simulink model "CC_CV"  (R2019a)
settings: Solver=ode23s  StartTime=0.0  StopTime=99  FixedStep=50e-6  RelTol=1e-8
libraries: powerlib x10, simulink x8
settings Model: Creator=Soto Porras  LastModifiedBy=juanj
settings DataIOCC: ReturnWorkspaceOutputs=off
settings DebuggingCC: ArithmeticOperatorsInVariantConditions=warning

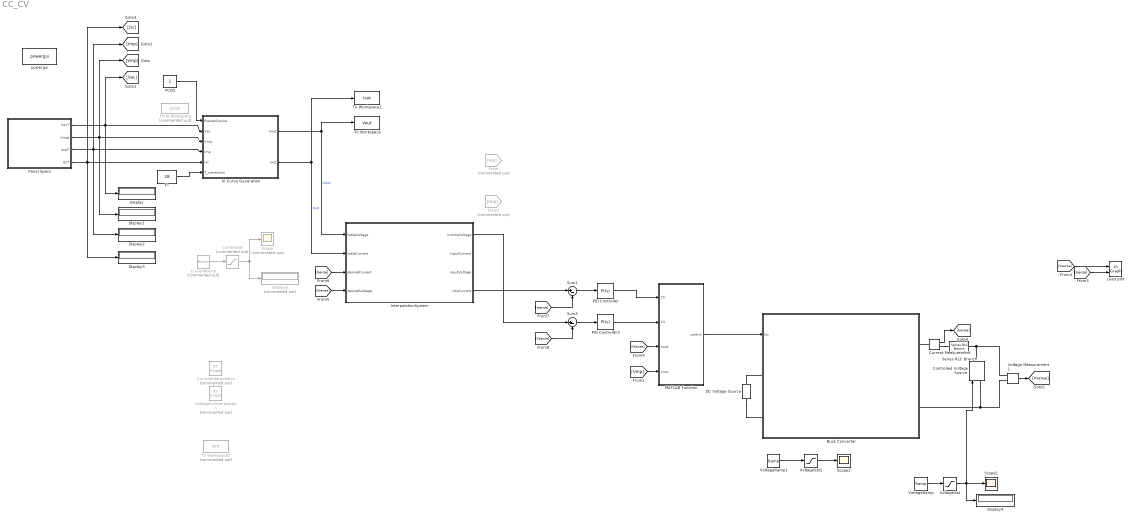
== system CC_CV ==
  Buck Converter : Subsystem
  Controlled Voltage Source : powerlib/Electrical Sources/Controlled Voltage Source  Initialize=off  Source_Type=DC  Amplitude=0  Phase=0  Frequency=0  Measurements=None
      settings: SourceProductName=Simscape Electrical
  Current Measurement : powerlib/Measurements/Current Measurement  PhasorSimulation=off  OutputType=Complex  PSBequivalent=0
      settings: SourceProductName=Simscape Electrical
  CurrentInterpolation : simulink/Sinks/XY Graph  Commented=on  xmin=0  xmax=6  ymin=0  ymax=2  st=-1
  CurrentRamp : simulink/Sources/Ramp  Commented=on  slope=0.015603  start=0  InitialOutput=0
  CurrentSat : Saturate  Commented=on  UpperLimit=1.5603  LowerLimit=0
  DC Voltage Source : powerlib/Electrical Sources/DC Voltage Source  Amplitude=15  Measurements=None
      settings: SourceProductName=Simscape Electrical
  Display{,1..4} (5 alike) : Display
  Display5 : Display  Commented=on
  From : From  Commented=on  GotoTag=Voc
  From Workspace : FromWorkspace  Commented=on  VariableName=pcos  SampleTime=0
  From2 : From  Commented=on  GotoTag=Imp
  IV Curve Generation : Subsystem  mask(Panel I-V Curve Calculation){ValueVocComp=0.0062, ValueVmpComp=0.0067}
      mask prompts: ValueVocComp "Voc Temperature Correction (V)"; ValueVmpComp "Vmp Temperature Correction (V)"
      mask help:
      | This module calculates the panel IV curve using the next panel parameters:
      | 1. Voc
      | 2. Vmp
      | 3. Imp
      | 4. Isc
      |
      | It applies:
      | 1. Correction to current parameters (Isc and Imp) using a pseudo cosine that varies depending on the angle of the perpendicular CubeSat face and the sun's incident radiation.
      | 2. Correction to voltage parameters (Voc and Vmp) using the panel datasheet voltage losses, given in V by the user.
      mask TypeOptions ValueVocComp: Voc_comp/Value
      mask TypeOptions ValueVmpComp: Vmp_comp/Value
      mask Display: image('IV_curve.png');
  InterpolationSystem : Subsystem
  Load plot : simulink/Sinks/XY Graph  xmin=0  xmax=6  ymin=0  ymax=2  st=-1
  MATLAB Function : MATLAB Function  TreatAsAtomicUnit=on
  PCOS : Constant
  PID Controller : simulink/Continuous/PID Controller  Controller=PI  Form=Parallel  TimeDomain=Continuous-time  SampleTime=0.00005  IntegratorMethod=Trapezoidal  FilterMethod=Forward Euler  ControllerParametersSource=internal  P=20  I=0.5  D=0  UseFilter=on  N=100  TunerSelectOption=Frequency Response Based  InitialConditionSource=internal  InitialConditionForIntegrator=0  InitialConditionForFilter=0  DifferentiatorICPrevScaledInput=0  ExternalReset=none  TrackingMode=off  Kt=1  LimitOutput=off  UpperSaturationLimit=inf  LowerSaturationLimit=-inf  LinearizeAsGain=on  AntiWindupMode=none  Kb=1  POutMin=[]  POutMax=[]  IOutMin=[]  IOutMax=[]  DOutMin=[]  DOutMax=[]  NOutMin=[]  NOutMax=[]  SumOutMin=[]  SumOutMax=[]  SaturationOutMin=[]  SaturationOutMax=[]  PParamMin=[]  PParamMax=[]  IParamMin=[]  IParamMax=[]  DParamMin=[]  DParamMax=[]  NParamMin=[]  NParamMax=[]  KbParamMin=[]  KbParamMax=[]  KtParamMin=[]  KtParamMax=[]  KbOutMin=[]  KbOutMax=[]  KtOutMin=[]  KtOutMax=[]  IntegratorOutMin=[]  IntegratorOutMax=[]  FilterOutMin=[]  FilterOutMax=[]  SumI1OutMin=[]  SumI1OutMax=[]  SumI2OutMin=[]  SumI2OutMax=[]  SumI3OutMin=[]  SumI3OutMax=[]  SumI4OutMin=[]  SumI4OutMax=[]  SumDOutMin=[]  SumDOutMax=[]  DifferentiatorOutMin=[]  DifferentiatorOutMax=[]  FilterDiffOutCoefMin=[]  FilterDiffOutCoefMax=[]  ReciprocalOutMin=[]  ReciprocalOutMax=[]  SumDenOutMin=[]  SumDenOutMax=[]  SumNumOutMin=[]  SumNumOutMax=[]  DivideOutMin=[]  DivideOutMax=[]  IntegratorContinuousStateAttributes=''  IntegratorStateMustResolveToSignalObject=off  IntegratorRTWStateStorageClass=Auto  FilterContinuousStateAttributes=''  FilterStateMustResolveToSignalObject=off  FilterRTWStateStorageClass=Auto  ParallelPVariant=InternalParameters  IdealPVariant=Disabled  IVariant=InternalParameters  DVariant=Disabled  IntegratorVariant=Continuous  SatVariant=Disabled  AWVariant=Passthrough  PCopyVariant=Disabled  TRVariant=Disabled  FdbkBlocksVariant=Forward  IdealPFdbkVariant=Disabled  SatFdbkVariant=Disabled  DerivativeFilterVariant=Disabled  NVariant=Disabled  NCopyVariant=Disabled_SignalSpec  FilterICVariant=Disabled  IntegratorICVariant=InternalICs  ExternalResetVariant=Disabled  TRSumVariant=Passthrough  SumFdbkVariant=Disabled  SumVariant=Sum_PI
  PID Controller2 : simulink/Continuous/PID Controller  Controller=PI  Form=Parallel  TimeDomain=Continuous-time  SampleTime=0.00005  IntegratorMethod=Trapezoidal  FilterMethod=Forward Euler  ControllerParametersSource=internal  P=20  I=0.01  D=0  UseFilter=on  N=100  TunerSelectOption=Frequency Response Based  InitialConditionSource=internal  InitialConditionForIntegrator=0  InitialConditionForFilter=0  DifferentiatorICPrevScaledInput=0  ExternalReset=none  TrackingMode=off  Kt=1  LimitOutput=off  UpperSaturationLimit=inf  LowerSaturationLimit=-inf  LinearizeAsGain=on  AntiWindupMode=none  Kb=1  POutMin=[]  POutMax=[]  IOutMin=[]  IOutMax=[]  DOutMin=[]  DOutMax=[]  NOutMin=[]  NOutMax=[]  SumOutMin=[]  SumOutMax=[]  SaturationOutMin=[]  SaturationOutMax=[]  PParamMin=[]  PParamMax=[]  IParamMin=[]  IParamMax=[]  DParamMin=[]  DParamMax=[]  NParamMin=[]  NParamMax=[]  KbParamMin=[]  KbParamMax=[]  KtParamMin=[]  KtParamMax=[]  KbOutMin=[]  KbOutMax=[]  KtOutMin=[]  KtOutMax=[]  IntegratorOutMin=[]  IntegratorOutMax=[]  FilterOutMin=[]  FilterOutMax=[]  SumI1OutMin=[]  SumI1OutMax=[]  SumI2OutMin=[]  SumI2OutMax=[]  SumI3OutMin=[]  SumI3OutMax=[]  SumI4OutMin=[]  SumI4OutMax=[]  SumDOutMin=[]  SumDOutMax=[]  DifferentiatorOutMin=[]  DifferentiatorOutMax=[]  FilterDiffOutCoefMin=[]  FilterDiffOutCoefMax=[]  ReciprocalOutMin=[]  ReciprocalOutMax=[]  SumDenOutMin=[]  SumDenOutMax=[]  SumNumOutMin=[]  SumNumOutMax=[]  DivideOutMin=[]  DivideOutMax=[]  IntegratorContinuousStateAttributes=''  IntegratorStateMustResolveToSignalObject=off  IntegratorRTWStateStorageClass=Auto  FilterContinuousStateAttributes=''  FilterStateMustResolveToSignalObject=off  FilterRTWStateStorageClass=Auto  ParallelPVariant=InternalParameters  IdealPVariant=Disabled  IVariant=InternalParameters  DVariant=Disabled  IntegratorVariant=Continuous  SatVariant=Disabled  AWVariant=Passthrough  PCopyVariant=Disabled  TRVariant=Disabled  FdbkBlocksVariant=Forward  IdealPFdbkVariant=Disabled  SatFdbkVariant=Disabled  DerivativeFilterVariant=Disabled  NVariant=Disabled  NCopyVariant=Disabled_SignalSpec  FilterICVariant=Disabled  IntegratorICVariant=InternalICs  ExternalResetVariant=Disabled  TRSumVariant=Passthrough  SumFdbkVariant=Disabled  SumVariant=Sum_PI
  Panel Specs : Subsystem  mask(Solar Panel Specifications){Voc=2.690, Vmp=2.409, Imp=0.5029, Isc=0.5196, SerialGain=2, ParallelGain=3}
      mask prompts: SerialGain "Serial"; ParallelGain "Parallel"
      mask help: Inputs solar panel electrical specifications, temperature and array distribution.
      mask TypeOptions Voc: Voc/Value
      mask TypeOptions Vmp: Vmp/Value
      mask TypeOptions Imp: Imp/Value
      mask TypeOptions Isc: Isc/Value
      mask TypeOptions SerialGain: Gain/Gain | Gain1/Gain
      mask TypeOptions ParallelGain: Gain2/Gain | Gain3/Gain
      mask DialogControl Container3 Prompt: Panel Array
      mask Display: image('solar_panel.png');
  Scope : Scope  Commented=on
  Scope1 : Scope
  Scope2 : Scope
  Series RLC Branch : powerlib/Elements/Series RLC Branch  LConnTagsString=__new0  RConnTagsString=__new0  BranchType=R  Resistance=1e-5  Inductance=1e-3  SetiL0=off  InitialCurrent=0  Capacitance=1e-6  Setx0=off  InitialVoltage=0  Measurements=None
      settings: SourceProductName=Simscape Electrical
  Sum1 : Sum  Inputs=|+-
  Sum3 : Sum  Inputs=|+-
  To Workspace : ToWorkspace  VariableName=Vout  SaveFormat=Structure With Time  SampleTime=-1
  To Workspace1 : ToWorkspace  VariableName=Iout  SaveFormat=Structure With Time  SampleTime=-1
  To Workspace2 : ToWorkspace  Commented=on  VariableName=Vint  SaveFormat=Structure With Time  SampleTime=-1
  T° : Constant  Value=28
  Voltage Measurement1 : powerlib/Measurements/Voltage Measurement  PhasorSimulation=off  OutputType=Complex  PSBequivalent=0
      settings: SourceProductName=Simscape Electrical
  VoltageInvInterpolation : simulink/Sinks/XY Graph  Commented=on  xmin=0  xmax=6  ymin=0  ymax=2  st=-1
  VoltageRamp : simulink/Sources/Ramp  slope=0.0538  start=0  InitialOutput=0
  VoltageRamp1 : simulink/Sources/Ramp  slope=0.0538  start=0  InitialOutput=0
  VoltageSat : Saturate  UpperLimit=5.37  LowerLimit=0.1
  VoltageSat1 : Saturate  UpperLimit=5.38  LowerLimit=0.1
  powergui : powerlib/powergui  Priority=1  SimulationMode=Continuous  SampleTime=50e-6  frequency=60  Iterations=50  frequencyindice=0  Pbase=100e6  ErrMax=1e-4  UnitsV=kV  UnitsW=MW  buscounter=0  FunctionMessages=off  echomessages=off  EnableUseOfTLC=off  CurrentSourceSwitches=off  DisableSnubberDevices=off  DisableRonSwitches=off  DisableVfSwitches=off  DisplayEquations=off  AutomaticDiscreteSolvers=off  SolverType=Tustin/Backward Euler (TBE)  Interpol=off  ExternalGateDelay=off  methode=off  Ts=100  x0status=blocks  SPID=on  SwTol=0  HookPort=off  NonlinearTolerance=0  nMaxIteration=15  ContinueOnMaxIteration=off  RestoreLinks=warning  ResistiveCurrentMeasurement=off  Frange=[0:2:500]  Ylog=off  Xlog=on  ShowGrid=off  save=off  variable=ZData  structure=0  ZoomFFT=off  StartTime=0.0  cycles=1  DisplayStyle=1  fundamental=60  FreqAxis=off  MaxFrequency=1000  frequencyindicesteady=1  RmsSteady=1  display=off
      settings: SourceProductName=Simscape Electrical
  wires:
  Panel Specs/1(VocT) -> [Voc], Display/1, IV Curve Generation/2(Voc)
  Panel Specs/2(Vmpt) -> [Vmp], Display1/1, IV Curve Generation/3(Vmp)
  Panel Specs/3(ImpT) -> [Imp], Display2/1, IV Curve Generation/4(Imp)
  Panel Specs/4(IscT) -> [Isc], Display3/1, IV Curve Generation/5(Isc)
  CurrentRamp/1 -> CurrentSat/1
  IV Curve Generation/1(Vout) -> InterpolationSystem/1(tableVoltage), To Workspace/1  "Vout"
  IV Curve Generation/2(Iout) -> To Workspace1/1, InterpolationSystem/2(tableCurrent)  "Iout"
  CurrentSat/1 -> Display5/1, Scope/1
  T°/1 -> IV Curve Generation/6(T_correction)
  Sum1/1 -> PID Controller/1
  VoltageRamp/1 -> VoltageSat/1
  VoltageSat/1 -> Controlled Voltage Source/1, Scope1/1, Display4/1
  Voltage Measurement1/1 -> [Vsense]
  Current Measurement/1 -> [Isense]
  VoltageRamp1/1 -> VoltageSat1/1
  VoltageSat1/1 -> Scope2/1
  InterpolationSystem/4(intpCurrent) -> Sum1/1
  PID Controller/1 -> MATLAB Function/1(CC)
  MATLAB Function/1(control) -> Buck Converter/1(Dc)
  PID Controller2/1 -> MATLAB Function/2(CV)
  Sum3/1 -> PID Controller2/1
  InterpolationSystem/1(invIntpVoltage) -> Sum3/1
  [Isense] -> Load plot/2
  [Vsense] -> Load plot/1
  [Vsense] -> InterpolationSystem/4(desiredVotlage)
  [Isense] -> InterpolationSystem/3(desiredCurrent)
  [Isense] -> Sum1/2
  [Vsense] -> Sum3/2
  [Vsense] -> MATLAB Function/3(Vout)
  [Vmp] -> MATLAB Function/4(Vmp)
  PCOS/1 -> IV Curve Generation/1(PseudoCosine)
  connections:
  DC Voltage Source/RConn1 -- Buck Converter/LConn1
  DC Voltage Source/LConn1 -- Buck Converter/LConn2
  Voltage Measurement1/LConn2 -- Controlled Voltage Source/LConn1 -- Buck Converter/RConn2
  Series RLC Branch/LConn1 -- Voltage Measurement1/LConn1 -- Controlled Voltage Source/RConn1
  Current Measurement/LConn1 -- Buck Converter/RConn1
  Current Measurement/RConn1 -- Series RLC Branch/RConn1

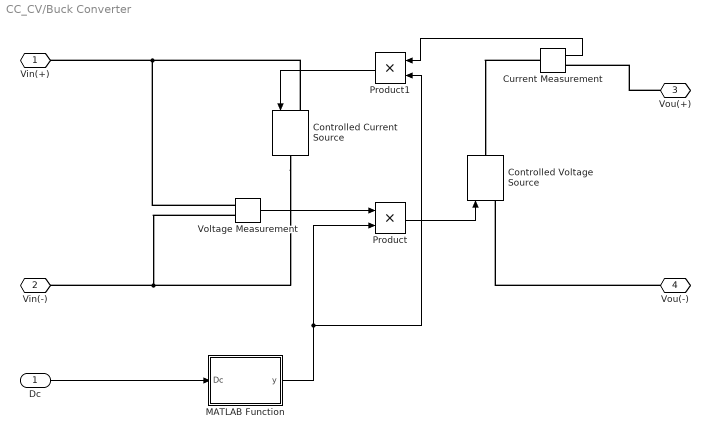
== system CC_CV/Buck Converter ==
  Dc : Inport
  Controlled Current Source : powerlib/Electrical Sources/Controlled Current Source  Initialize=off  Source_Type=DC  Amplitude=0  Phase=0  Frequency=0  Measurements=None
      settings: SourceProductName=Simscape Electrical
  Controlled Voltage Source : powerlib/Electrical Sources/Controlled Voltage Source  Initialize=off  Source_Type=DC  Amplitude=0  Phase=0  Frequency=0  Measurements=None
      settings: SourceProductName=Simscape Electrical
  Current Measurement : powerlib/Measurements/Current Measurement  PhasorSimulation=off  OutputType=Complex  PSBequivalent=0
      settings: SourceProductName=Simscape Electrical
  MATLAB Function : MATLAB Function  TreatAsAtomicUnit=on
  Product : Product
  Product1 : Product
  Voltage Measurement : powerlib/Measurements/Voltage Measurement  PhasorSimulation=off  OutputType=Complex  PSBequivalent=0
      settings: SourceProductName=Simscape Electrical
  Vin(+) : PMIOPort  Side=Left
  Vin(-) : PMIOPort  Port=2  Side=Left
  Vou(+) : PMIOPort  Port=3  Side=Right
  Vou(-) : PMIOPort  Port=4  Side=Right
  wires:
  Product/1 -> Controlled Voltage Source/1
  Current Measurement/1 -> Product1/1
  Product1/1 -> Controlled Current Source/1
  MATLAB Function/1(y) -> Product1/2, Product/2
  Voltage Measurement/1 -> Product/1
  Dc/1 -> MATLAB Function/1(Dc)
  connections:
  Controlled Current Source/RConn1 -- Voltage Measurement/LConn2 -- Vin(-)/RConn1
  Vou(-)/RConn1 -- Controlled Voltage Source/LConn1
  Current Measurement/LConn1 -- Controlled Voltage Source/RConn1
  Controlled Current Source/LConn1 -- Voltage Measurement/LConn1 -- Vin(+)/RConn1
  Vou(+)/RConn1 -- Current Measurement/RConn1

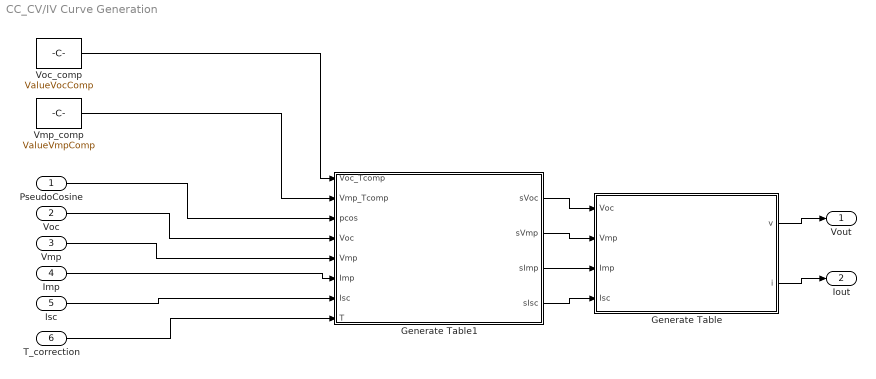
== system CC_CV/IV Curve Generation ==
  PseudoCosine : Inport
  Voc : Inport  Port=2
  Vmp : Inport  Port=3
  Imp : Inport  Port=4
  Isc : Inport  Port=5
  T_correction : Inport  Port=6
  Generate Table : MATLAB Function  TreatAsAtomicUnit=on
  Generate Table1 : MATLAB Function  TreatAsAtomicUnit=on
  Vmp_comp : Constant  Value=ValueVmpComp
  Voc_comp : Constant  Value=ValueVocComp
  Vout : Outport
  Iout : Outport  Port=2
  wires:
  Isc/1 -> Generate Table1/7(Isc)
  Generate Table1/4(sIsc) -> Generate Table/4(Isc)
  Voc_comp/1 -> Generate Table1/1(Voc_Tcomp)
  Generate Table/1(v) -> Vout/1
  T_correction/1 -> Generate Table1/8(T)
  Generate Table1/2(sVmp) -> Generate Table/2(Vmp)
  Voc/1 -> Generate Table1/4(Voc)
  Generate Table1/3(sImp) -> Generate Table/3(Imp)
  Imp/1 -> Generate Table1/6(Imp)
  Generate Table1/1(sVoc) -> Generate Table/1(Voc)
  Vmp/1 -> Generate Table1/5(Vmp)
  Generate Table/2(i) -> Iout/1
  Vmp_comp/1 -> Generate Table1/2(Vmp_Tcomp)
  PseudoCosine/1 -> Generate Table1/3(pcos)

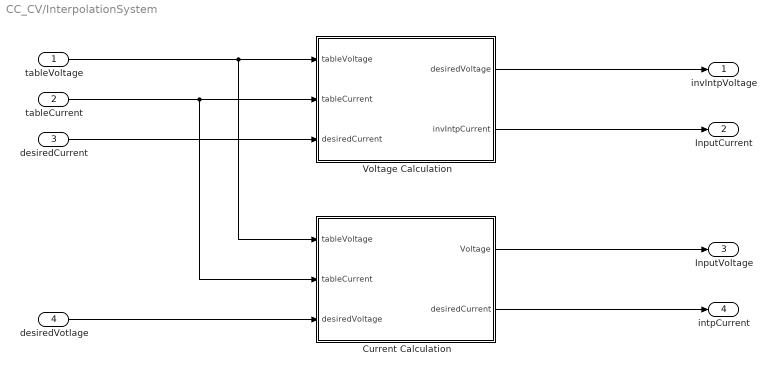
== system CC_CV/InterpolationSystem ==
  tableVoltage : Inport
  tableCurrent : Inport  Port=2
  desiredCurrent : Inport  Port=3
  desiredVotlage : Inport  Port=4
  Current Calculation : MATLAB Function  TreatAsAtomicUnit=on
  Voltage Calculation : MATLAB Function  TreatAsAtomicUnit=on
  invIntpVoltage : Outport
  InputCurrent : Outport  Port=2
  InputVoltage : Outport  Port=3
  intpCurrent : Outport  Port=4
  wires:
  Current Calculation/1(Voltage) -> InputVoltage/1
  Voltage Calculation/1(desiredVoltage) -> invIntpVoltage/1
  tableVoltage/1 -> Voltage Calculation/1(tableVoltage), Current Calculation/1(tableVoltage)
  Current Calculation/2(desiredCurrent) -> intpCurrent/1
  tableCurrent/1 -> Voltage Calculation/2(tableCurrent), Current Calculation/2(tableCurrent)
  Voltage Calculation/2(invIntpCurrent) -> InputCurrent/1
  desiredCurrent/1 -> Voltage Calculation/3(desiredCurrent)
  desiredVotlage/1 -> Current Calculation/3(desiredVoltage)

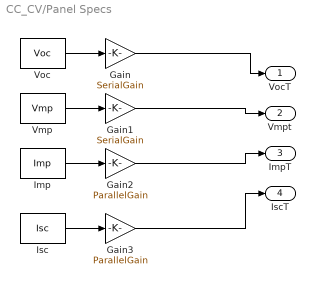
== system CC_CV/Panel Specs ==
  Gain : Gain  Gain=SerialGain
  Gain1 : Gain  Gain=SerialGain
  Gain2 : Gain  Gain=ParallelGain
  Gain3 : Gain  Gain=ParallelGain
  Imp : Constant  Value=Imp
  Isc : Constant  Value=Isc
  Vmp : Constant  Value=Vmp
  Voc : Constant  Value=Voc
  VocT : Outport
  Vmpt : Outport  Port=2
  ImpT : Outport  Port=3
  IscT : Outport  Port=4
  wires:
  Isc/1 -> Gain3/1
  Vmp/1 -> Gain1/1
  Gain/1 -> VocT/1
  Imp/1 -> Gain2/1
  Gain2/1 -> ImpT/1
  Gain3/1 -> IscT/1
  Voc/1 -> Gain/1
  Gain1/1 -> Vmpt/1

== matlab function CC_CV/Buck Converter/MATLAB Function ==
  data: Dc input; y output
function y = M(Dc)
y = Dc;

== matlab function CC_CV/InterpolationSystem/Voltage Calculation ==
  data: desiredVoltage output; tableVoltage input; tableCurrent input; invIntpCurrent output; desiredCurrent input
function [desiredVoltage, invIntpCurrent] = CurrentInverseInterpolation(tableVoltage, tableCurrent, desiredCurrent)
    
    % Apply inverse interpolation on ampere ramp values
    n = 1024;
    v = 0;
    %i = 1023;
    for j = 1 : n - 1
        i = 1024 - j;
        if(desiredCurrent < tableCurrent(i))
           v = tableVoltage(i) + (tableVoltage(i+1)-tableVoltage(i))*((desiredCurrent - tableCurrent(i))/(tableCurrent(i+1) - tableCurrent(i)));
           break;
        end
    end
     desiredVoltage = v;
     invIntpCurrent = desiredCurrent;
    
end

== matlab function CC_CV/IV Curve Generation/Generate Table ==
  data: Voc input; Vmp input; Imp input; Isc input; v output; i output
function [v,i] = generate_table(Voc, Vmp, Imp, Isc)
Rs = ( Voc - Vmp ) / Imp;
a = ( Vmp * ( 1 + ( Rs*Isc ) / Voc ) + Rs*( Imp - Isc ) ) / Voc;
N = log( 2 - 2^a) / log ( Imp / Isc );
i=zeros(1024,1);
v=zeros(1024,1);
for x = 1:1024
    I = (x * Isc) / 1023.0;
    V = Voc * log( 2 - ( ( I / Isc ) ^ N ) );
    V = V / log( 2 );
    V = V - Rs * ( I - Isc );
    V = V / ( 1 + ( ( Rs * Isc) / Voc) );
    P = V * I;
    v(x) = V;
    i(x) = I;
end
v = flip(v);
i = flip(i);

== matlab function CC_CV/InterpolationSystem/Current Calculation ==
  data: Voltage output; desiredCurrent output; tableVoltage input; tableCurrent input; desiredVoltage input
function [Voltage, desiredCurrent] = VoltageInterpolation(tableVoltage, tableCurrent, desiredVoltage)
    
    % Apply interpolation on voltage ramp values
    n = 1023;
    c = 0;
    for j = 1 : n + 1
        i = j;
        if(desiredVoltage < tableVoltage(i))
           c = tableCurrent(i) + ...
               (tableCurrent(i-1)-tableCurrent(i))*...
               ((desiredVoltage - tableVoltage(i))/(tableVoltage(i-1) - tableVoltage(i)));
           break;
        end
    end

    
%     for i = 1 : n
%         vi = tableVoltage(i);
%         for j = 1 : n
%             if(j ~= i)
%                 vi = vi*((y-tableCurrent(j))/(tableCurrent(i) - tableCurrent(j)));
%             end
%         end
%         invIntpVoltageHelper = invIntpVoltageHelper + vi;
%     end
% 
     desiredCurrent = c;
     Voltage = desiredVoltage;
    
end

== matlab function CC_CV/MATLAB Function ==
  data: CC input; control output; CV input; Vout input; Vmp input
function control = CC_CV(CC,CV,Vout,Vmp)

    if Vout >= Vmp
        control = CV;
    else 
        control = CC;
end

== matlab function CC_CV/IV Curve Generation/Generate Table1 ==
  data: Voc_Tcomp input; Vmp_Tcomp input; pcos input; Voc input; Vmp input; Imp input; Isc input; sVoc output; sVmp output; sImp output; sIsc output; T input
function [sVoc, sVmp, sImp, sIsc] = scalevars(Voc_Tcomp, Vmp_Tcomp, pcos, Voc, Vmp, Imp, Isc, T)
sVoc = Voc-(T*Voc_Tcomp);
sVmp = Vmp-(T*Vmp_Tcomp);
sImp = pcos * Imp;
sIsc = pcos * Isc;
